simulink model "linear_model_Quadcopter_02_09_2019"  (R2019a)
settings: Solver=VariableStepAuto  StartTime=0.0  StopTime=inf  RelTol=1e-3
undefined symbols (not defined in the file): DiscIntNeverNeededParam
libraries: simulink x3
settings Model: Creator=DINESH  LastModifiedBy=DINESH
settings DataIOCC: ReturnWorkspaceOutputs=off
settings DebuggingCC: PregeneratedLibrarySubsystemCodeDiagnostic=none  ArithmeticOperatorsInVariantConditions=warning
settings SFSimCC: SimUseLocalCustomCode=off
settings RTWCC: RTWUseLocalCustomCode=off

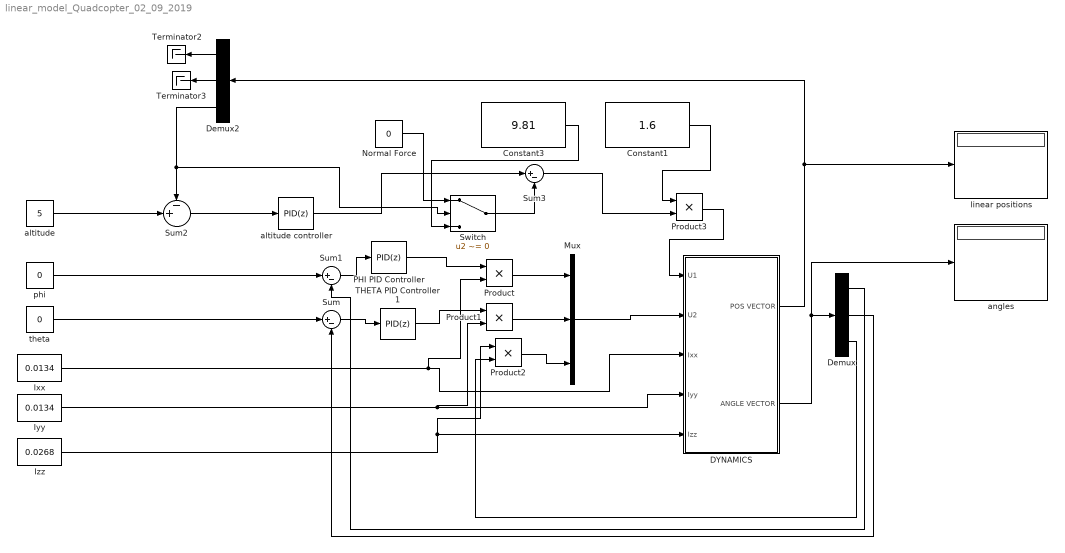
== system linear_model_Quadcopter_02_09_2019 ==
  Constant1 : Constant  Value=1.6
  Constant3 : Constant  Value=9.81
  "DYNAMICS " : Subsystem
  Demux : Demux  Outputs=3
  Demux2 : Demux  Outputs=3
  Ixx : Constant  Value=0.0134
  Iyy : Constant  Value=0.0134
  Izz : Constant  Value=0.0268
  Mux : Mux  Inputs=3
  "Normal Force " : Constant  Value=0
  PHI PID Controller : simulink/Continuous/PID Controller  Controller=PID  Form=Parallel  TimeDomain=Discrete-time  SampleTime=-1  IntegratorMethod=Forward Euler  FilterMethod=Forward Euler  ControllerParametersSource=internal  P=0.0266430851222438  I=0.00015614484496637  D=0.943041683036594  UseFilter=on  N=4.99178863294947  TunerSelectOption=Transfer Function Based (PID Tuner App)  InitialConditionSource=internal  InitialConditionForIntegrator=0  InitialConditionForFilter=0  DifferentiatorICPrevScaledInput=0  ExternalReset=none  TrackingMode=off  Kt=1  LimitOutput=off  UpperSaturationLimit=inf  LowerSaturationLimit=-inf  LinearizeAsGain=on  AntiWindupMode=none  Kb=1  POutMin=[]  POutMax=[]  IOutMin=[]  IOutMax=[]  DOutMin=[]  DOutMax=[]  NOutMin=[]  NOutMax=[]  SumOutMin=[]  SumOutMax=[]  SaturationOutMin=[]  SaturationOutMax=[]  PParamMin=[]  PParamMax=[]  IParamMin=[]  IParamMax=[]  DParamMin=[]  DParamMax=[]  NParamMin=[]  NParamMax=[]  KbParamMin=[]  KbParamMax=[]  KtParamMin=[]  KtParamMax=[]  KbOutMin=[]  KbOutMax=[]  KtOutMin=[]  KtOutMax=[]  IntegratorOutMin=[]  IntegratorOutMax=[]  FilterOutMin=[]  FilterOutMax=[]  SumI1OutMin=[]  SumI1OutMax=[]  SumI2OutMin=[]  SumI2OutMax=[]  SumI3OutMin=[]  SumI3OutMax=[]  SumI4OutMin=[]  SumI4OutMax=[]  SumDOutMin=[]  SumDOutMax=[]  DifferentiatorOutMin=[]  DifferentiatorOutMax=[]  FilterDiffOutCoefMin=[]  FilterDiffOutCoefMax=[]  ReciprocalOutMin=[]  ReciprocalOutMax=[]  SumDenOutMin=[]  SumDenOutMax=[]  SumNumOutMin=[]  SumNumOutMax=[]  DivideOutMin=[]  DivideOutMax=[]  IntegratorContinuousStateAttributes=''  IntegratorStateMustResolveToSignalObject=off  IntegratorRTWStateStorageClass=Auto  FilterContinuousStateAttributes=''  FilterStateMustResolveToSignalObject=off  FilterRTWStateStorageClass=Auto  ParallelPVariant=InternalParameters  IdealPVariant=Disabled  IVariant=InternalParameters  DVariant=InternalParameters  IntegratorVariant=Discrete  SatVariant=Disabled  AWVariant=Passthrough  PCopyVariant=Disabled  TRVariant=Disabled  FdbkBlocksVariant=Forward  IdealPFdbkVariant=Disabled  SatFdbkVariant=Disabled  DerivativeFilterVariant=ForwardEulerFilter  NVariant=InternalParameters  NCopyVariant=Disabled  FilterICVariant=InternalICsFilter  IntegratorICVariant=InternalICs  ExternalResetVariant=Disabled  TRSumVariant=Passthrough  SumFdbkVariant=Disabled  SumVariant=Sum_PID
  Product{,1..3} (4 alike) : Product
  Sum : Sum  Inputs=|+-
  Sum1 : Sum  Inputs=|+-
  Sum2 : Sum  Inputs=-+|
  Sum3 : Sum  Inputs=|+-
  Switch : Switch  Criteria=u2 ~= 0
  THETA PID Controller1 : simulink/Continuous/PID Controller  Controller=PID  Form=Parallel  TimeDomain=Discrete-time  SampleTime=-1  IntegratorMethod=Forward Euler  FilterMethod=Forward Euler  ControllerParametersSource=internal  P=0.0148409171786849  I=6.52468600062285e-05  D=0.749377908750691  UseFilter=on  N=8.96007490651367  TunerSelectOption=Transfer Function Based (PID Tuner App)  InitialConditionSource=internal  InitialConditionForIntegrator=0  InitialConditionForFilter=0  DifferentiatorICPrevScaledInput=0  ExternalReset=none  TrackingMode=off  Kt=1  LimitOutput=off  UpperSaturationLimit=inf  LowerSaturationLimit=-inf  LinearizeAsGain=on  AntiWindupMode=none  Kb=1  POutMin=[]  POutMax=[]  IOutMin=[]  IOutMax=[]  DOutMin=[]  DOutMax=[]  NOutMin=[]  NOutMax=[]  SumOutMin=[]  SumOutMax=[]  SaturationOutMin=[]  SaturationOutMax=[]  PParamMin=[]  PParamMax=[]  IParamMin=[]  IParamMax=[]  DParamMin=[]  DParamMax=[]  NParamMin=[]  NParamMax=[]  KbParamMin=[]  KbParamMax=[]  KtParamMin=[]  KtParamMax=[]  KbOutMin=[]  KbOutMax=[]  KtOutMin=[]  KtOutMax=[]  IntegratorOutMin=[]  IntegratorOutMax=[]  FilterOutMin=[]  FilterOutMax=[]  SumI1OutMin=[]  SumI1OutMax=[]  SumI2OutMin=[]  SumI2OutMax=[]  SumI3OutMin=[]  SumI3OutMax=[]  SumI4OutMin=[]  SumI4OutMax=[]  SumDOutMin=[]  SumDOutMax=[]  DifferentiatorOutMin=[]  DifferentiatorOutMax=[]  FilterDiffOutCoefMin=[]  FilterDiffOutCoefMax=[]  ReciprocalOutMin=[]  ReciprocalOutMax=[]  SumDenOutMin=[]  SumDenOutMax=[]  SumNumOutMin=[]  SumNumOutMax=[]  DivideOutMin=[]  DivideOutMax=[]  IntegratorContinuousStateAttributes=''  IntegratorStateMustResolveToSignalObject=off  IntegratorRTWStateStorageClass=Auto  FilterContinuousStateAttributes=''  FilterStateMustResolveToSignalObject=off  FilterRTWStateStorageClass=Auto  ParallelPVariant=InternalParameters  IdealPVariant=Disabled  IVariant=InternalParameters  DVariant=InternalParameters  IntegratorVariant=Discrete  SatVariant=Disabled  AWVariant=Passthrough  PCopyVariant=Disabled  TRVariant=Disabled  FdbkBlocksVariant=Forward  IdealPFdbkVariant=Disabled  SatFdbkVariant=Disabled  DerivativeFilterVariant=ForwardEulerFilter  NVariant=InternalParameters  NCopyVariant=Disabled  FilterICVariant=InternalICsFilter  IntegratorICVariant=InternalICs  ExternalResetVariant=Disabled  TRSumVariant=Passthrough  SumFdbkVariant=Disabled  SumVariant=Sum_PID
  Terminator2 : Terminator
  Terminator3 : Terminator
  "altitude " : Constant  Value=5
  altitude controller : simulink/Continuous/PID Controller  Controller=PID  Form=Parallel  TimeDomain=Discrete-time  SampleTime=-1  IntegratorMethod=Forward Euler  FilterMethod=Forward Euler  ControllerParametersSource=internal  P=0.0216592919341655  I=9.09241902969596e-05  D=1.14542151097321  UseFilter=on  N=8.91621472154284  TunerSelectOption=Transfer Function Based (PID Tuner App)  InitialConditionSource=internal  InitialConditionForIntegrator=0  InitialConditionForFilter=0  DifferentiatorICPrevScaledInput=0  ExternalReset=none  TrackingMode=off  Kt=1  LimitOutput=off  UpperSaturationLimit=inf  LowerSaturationLimit=-inf  LinearizeAsGain=on  AntiWindupMode=none  Kb=1  POutMin=[]  POutMax=[]  IOutMin=[]  IOutMax=[]  DOutMin=[]  DOutMax=[]  NOutMin=[]  NOutMax=[]  SumOutMin=[]  SumOutMax=[]  SaturationOutMin=[]  SaturationOutMax=[]  PParamMin=[]  PParamMax=[]  IParamMin=[]  IParamMax=[]  DParamMin=[]  DParamMax=[]  NParamMin=[]  NParamMax=[]  KbParamMin=[]  KbParamMax=[]  KtParamMin=[]  KtParamMax=[]  KbOutMin=[]  KbOutMax=[]  KtOutMin=[]  KtOutMax=[]  IntegratorOutMin=[]  IntegratorOutMax=[]  FilterOutMin=[]  FilterOutMax=[]  SumI1OutMin=[]  SumI1OutMax=[]  SumI2OutMin=[]  SumI2OutMax=[]  SumI3OutMin=[]  SumI3OutMax=[]  SumI4OutMin=[]  SumI4OutMax=[]  SumDOutMin=[]  SumDOutMax=[]  DifferentiatorOutMin=[]  DifferentiatorOutMax=[]  FilterDiffOutCoefMin=[]  FilterDiffOutCoefMax=[]  ReciprocalOutMin=[]  ReciprocalOutMax=[]  SumDenOutMin=[]  SumDenOutMax=[]  SumNumOutMin=[]  SumNumOutMax=[]  DivideOutMin=[]  DivideOutMax=[]  IntegratorContinuousStateAttributes=''  IntegratorStateMustResolveToSignalObject=off  IntegratorRTWStateStorageClass=Auto  FilterContinuousStateAttributes=''  FilterStateMustResolveToSignalObject=off  FilterRTWStateStorageClass=Auto  ParallelPVariant=InternalParameters  IdealPVariant=Disabled  IVariant=InternalParameters  DVariant=InternalParameters  IntegratorVariant=Discrete  SatVariant=Disabled  AWVariant=Passthrough  PCopyVariant=Disabled  TRVariant=Disabled  FdbkBlocksVariant=Forward  IdealPFdbkVariant=Disabled  SatFdbkVariant=Disabled  DerivativeFilterVariant=ForwardEulerFilter  NVariant=InternalParameters  NCopyVariant=Disabled  FilterICVariant=InternalICsFilter  IntegratorICVariant=InternalICs  ExternalResetVariant=Disabled  TRSumVariant=Passthrough  SumFdbkVariant=Disabled  SumVariant=Sum_PID
  "angles " : Display
  "linear positions " : Display
  phi : Constant  Value=0
  theta : Constant  Value=0
  wires:
  Mux/1 -> "DYNAMICS "/2(U2)
  "DYNAMICS "/2("ANGLE VECTOR ") -> "angles "/1, Demux/1
  Sum/1 -> THETA PID Controller1/1
  Sum1/1 -> PHI PID Controller/1
  Demux/2 -> Sum/2
  Demux/1 -> Sum1/2
  phi/1 -> Sum1/1
  theta/1 -> Sum/1
  Sum2/1 -> altitude controller/1
  Ixx/1 -> Product/2, "DYNAMICS "/3(Ixx)
  Iyy/1 -> Product1/2, "DYNAMICS "/4(Iyy)
  Izz/1 -> Product2/1, "DYNAMICS "/5(Izz)
  PHI PID Controller/1 -> Product/1
  THETA PID Controller1/1 -> Product1/1
  Demux/3 -> Product2/2
  Product2/1 -> Mux/3
  Product1/1 -> Mux/2
  Product/1 -> Mux/1
  "DYNAMICS "/1(POS VECTOR) -> Demux2/1, "linear positions "/1
  "altitude "/1 -> Sum2/2
  Demux2/1 -> Terminator2/1
  Demux2/2 -> Terminator3/1
  Constant3/1 -> Switch/3
  "Normal Force "/1 -> Switch/1
  Demux2/3 -> Switch/2, Sum2/1
  Switch/1 -> Sum3/2
  altitude controller/1 -> Sum3/1
  Constant1/1 -> Product3/1
  Sum3/1 -> Product3/2
  Product3/1 -> "DYNAMICS "/1(U1)

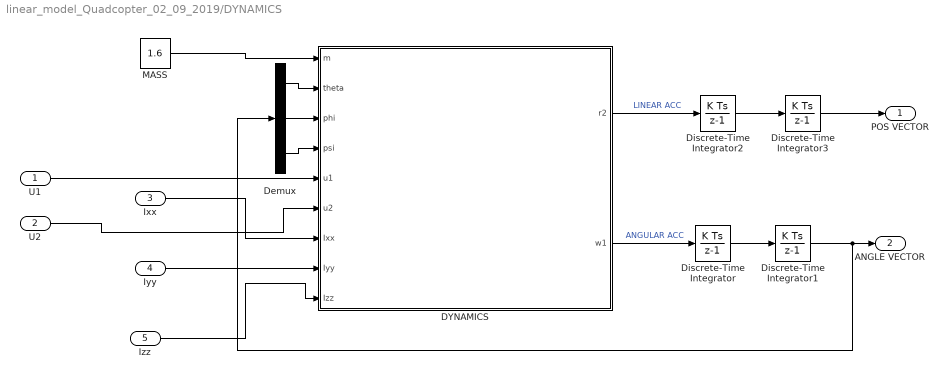
== system linear_model_Quadcopter_02_09_2019/DYNAMICS  ==
  U1 : Inport
  U2 : Inport  Port=2
  Ixx : Inport  Port=3
  Iyy : Inport  Port=4
  Izz : Inport  Port=5
  "DYNAMICS " : MATLAB Function  TreatAsAtomicUnit=on
  Demux : Demux  Outputs=3
  Discrete-Time Integrator{,1..3} (4 alike) : DiscreteIntegrator  SampleTime=-1  ICPrevOutput=DiscIntNeverNeededParam  ICPrevScaledInput=DiscIntNeverNeededParam
  "MASS " : Constant  Value=1.6
  POS VECTOR : Outport
  "ANGLE VECTOR " : Outport  Port=2
  wires:
  Demux/3 -> "DYNAMICS "/4(psi)
  Izz/1 -> "DYNAMICS "/9(Izz)
  Discrete-Time Integrator3/1 -> POS VECTOR/1
  Iyy/1 -> "DYNAMICS "/8(Iyy)
  Discrete-Time Integrator1/1 -> Demux/1, "ANGLE VECTOR "/1
  "DYNAMICS "/2(w1) -> Discrete-Time Integrator/1  "ANGULAR ACC"
  "DYNAMICS "/1(r2) -> Discrete-Time Integrator2/1  "LINEAR ACC"
  U2/1 -> "DYNAMICS "/6(u2)
  Ixx/1 -> "DYNAMICS "/7(Ixx)
  Demux/2 -> "DYNAMICS "/3(phi)
  "MASS "/1 -> "DYNAMICS "/1(m)
  Discrete-Time Integrator/1 -> Discrete-Time Integrator1/1
  Discrete-Time Integrator2/1 -> Discrete-Time Integrator3/1
  Demux/1 -> "DYNAMICS "/2(theta)
  U1/1 -> "DYNAMICS "/5(u1)

== matlab function linear_model_Quadcopter_02_09_2019/DYNAMICS /DYNAMICS  ==
  data: m input; r2 output size=[3,1]; theta input; phi input size=[1,1]; psi input; u1 input; u2 input; Ixx input; w1 output size=[3,1]; Iyy input; Izz input
function [r2 ,w1] = fcn(m,theta,phi,psi,u1,u2,Ixx,Iyy,Izz)
    I = [Ixx 0 0;
        0 Iyy 0 ;
        0 0 Izz];
    
    G = [0;0;-9.81];
    r2 = (1/m).*[cos(psi), -sin(psi) ,(phi*sin(psi)+theta*cos(psi));sin(psi), cos(psi), (-phi*cos(psi)+theta*sin(psi)) ;-theta ,phi ,1]  * [0;0;u1]  +G;

    
    w1 = inv(I)*u2;
    
    
    
    
    
end
